simulink model "Chemical_Akzo___Copy"  (Simulink 10.0)
settings: Solver=ode45  StartTime=0.0  StopTime=180  RelTol=1e-3  EnableMultiTasking=on
settings Model: Creator=UX31  LastModifiedBy=unknown
settings DataIOCC: LimitDataPoints=on
settings DebuggingCC: UnderspecifiedInitializationDetection=Simplified  MergeDetectMultiDrivingBlocksExec=error  SolverPrmCheckMsg=warning
settings GRTTargetCC: GeneratePreprocessorConditionals=Disable all  CombineOutputUpdateFcns=on  GRTInterface=off
settings ConfigComp: CovExternalEMLEnable=off  CovSFcnEnable=off

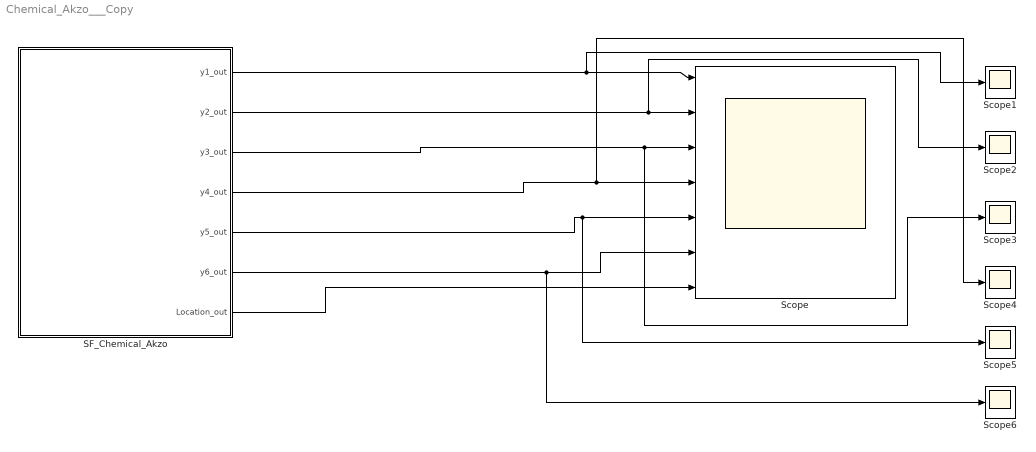
== system Chemical_Akzo___Copy ==
  SF_Chemical_Akzo : Stateflow chart  TreatAsAtomicUnit=on
  Scope : Scope  NumInputPorts=7
  Scope{1..6} (6 alike) : Scope
  wires:
  SF_Chemical_Akzo/1(y1_out) -> Scope1/1, Scope/1
  SF_Chemical_Akzo/2(y2_out) -> Scope2/1, Scope/2
  SF_Chemical_Akzo/3(y3_out) -> Scope3/1, Scope/3
  SF_Chemical_Akzo/4(y4_out) -> Scope4/1, Scope/4
  SF_Chemical_Akzo/5(y5_out) -> Scope5/1, Scope/5
  SF_Chemical_Akzo/6(y6_out) -> Scope6/1, Scope/6
  SF_Chemical_Akzo/7(Location_out) -> Scope/7

== stateflow chart SF_Chemical_Akzo ==
  settings: updateMethod=CONTINUOUS
  state Chemical_Akzo
    du:
    y1_dot=-2*k1*(y1^4)*(y2^0.5)+k2*y3*y4-k2/K*y1*y5-k3*y1*(y4^2);
    y2_dot=-0.5*k1*(y1^4)*(y2^0.5)-k3*y1*(y4^2)-0.5*k4*(y6^2)*(y2^0.5)+klA*(p_CO2/H-y2);
    y3_dot=k1*(y1^4)*(y2^0.5)-k2*y3*y4+(k2/K)*y1*y5;
    y4_dot= -k2*y3*y4+(k2/K)*y1*y5-2*k3*y1*(y4^2);
    y5_dot=k2*y3*y4-(k2/K)*y1*y5+k4*(y6^2)*(y2^0.5);
    y6_dot=Ks*(y4*(-2*k1*(y1^4)*(y2^0.5)+k2*y3*y4-k2/K*y1*y5-k3*y1*(y4^2))+y1*(-k2*y3*y4+(k2/K)*y1*y5-2*k3*y1*(y4^2)));
    y1_out=y1;
    y2_out=y2;
    y3_out=y3;
    y4_out=y4;
    y5_out=y5;
    y6_out=y6;
    Location_out =1;
  (default) -> Chemical_Akzo : {y1=0.444;y2=0.00123;y3=0;y4=0.007;y5=0;y6=0.35999964}
  data: y1 local double; y1_out output double; y2 local double; y2_out output double; y3 local double; y3_out output double; y4 local double; y4_out output double; y5 local double; y5_out output double; y6 local double; y6_out output double; Location_out output double; k1 constant double =18.7; k2 constant double =0.58; k3 constant double =0.09; k4 constant double =0.42; K constant double =34.4; klA constant double =3.3; Ks constant double =115.83; p_CO2 constant double =0.9; H constant double =737
  data y1 settings: updateMethod=SF_CONTINUOUS_TIME_DATA
  data y2 settings: updateMethod=SF_CONTINUOUS_TIME_DATA
  data y3 settings: updateMethod=SF_CONTINUOUS_TIME_DATA
  data y4 settings: updateMethod=SF_CONTINUOUS_TIME_DATA
  data y5 settings: updateMethod=SF_CONTINUOUS_TIME_DATA
  data y6 settings: updateMethod=SF_CONTINUOUS_TIME_DATA
